simulink model "MPC_test_SG"  (R2024b)
settings: Solver=FixedStepAuto  StartTime=0.0  StopTime=20  FixedStep=0.02  RelTol=1e-3
values from neighbouring files (symbols this model uses):
  Eff = fit(Js, Effs, 'poly9')    [SG01_Flight_Dynamics.m]    (also in SG01_Flight_Dynamics_original.m)
  T = rho*(Rpms_propeller/60)^2*diam^4*kt    [SG01_Flight_Dynamics.m]    (also in SG01_Flight_Dynamics_original.m)
undefined symbols (not defined in the file or in its folder): initial_P, initial_Pitch, initial_Q, initial_R, initial_ROLL, initial_uspeed, initial_vspeed, initial_wspeed, initial_YAW, initial_Z
libraries: mpclib x1, slpidlib x1
settings Model: Creator=Basile  LastModifiedBy=ricar
settings SolverCC: ConcurrentTasks=on  ZeroCrossAlgorithm=Adaptive  AlgebraicLoopSolver=TrustRegion  PositivePriorityOrder=on
settings DataIOCC: ExternalInput=getinputstruct(op_trim1)  InitialState=getstatestruct(op_trim1)  SaveOutput=off  DSMLogging=off  SaveTime=off  ReturnWorkspaceOutputs=off
settings OptimizationCC: BlockReduction=off  DefaultParameterBehavior=Inlined  UseDivisionForNetSlopeComputation=on  UseFloatMulNetSlope=on  OptimizeBlockIOStorage=off  BufferReuse=off  PassReuseOutputArgsThreshold=0  EfficientFloat2IntCast=on  OptimizeBlockOrder=speed  DifferentSizesBufferReuse=on
settings DebuggingCC: InheritedTsInSrcMsg=none  TasksWithSamePriorityMsg=none  ParameterTunabilityLossMsg=error  UniqueDataStoreMsg=error  ArithmeticOperatorsInVariantConditions=warning
settings HardwareCC: ProdBitPerLong=64  ProdLongLongMode=on  ProdHWDeviceType=Intel->x86-64 (Linux 64)
settings ModelReferenceCC: EnableRefExpFcnMdlSchedulingChecks=on
settings SFSimCC: SimUseLocalCustomCode=off  MATLABDynamicMemAlloc=off  CustomCodeUndefinedFunction=UseInterfaceOnly
settings RTWCC: Description=Simulink Real-Time  SystemTargetFile=slrealtime.tlc  TemplateMakefile=slrealtime_default_tmf  GenerateReport=on  RTWUseLocalCustomCode=off  Toolchain=Simulink Real-Time Toolchain  BuildConfiguration=Faster Runs  LaunchReport=on  CodeExecutionProfiling=on  TargetLang=C++  GPUComputeCapability=3.5  DLArmComputeVersion=19.05
settings CodeAppCC: ForceParamTrailComments=on  OperatorAnnotations=on
settings SimulinkRealTimeTargetCC: InstructionSetFMA=off  LogToMDFFile=off

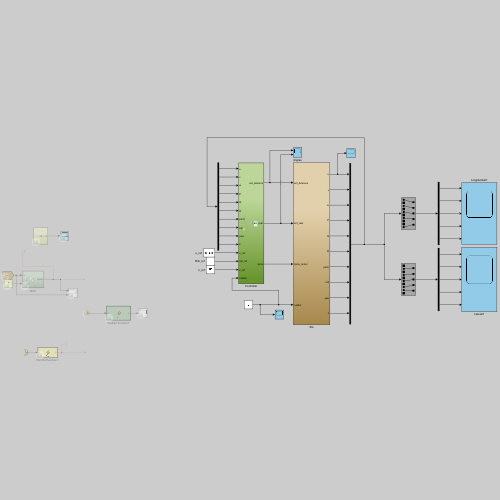
[thumbnail: Simulink's stored preview of the top-level diagram]
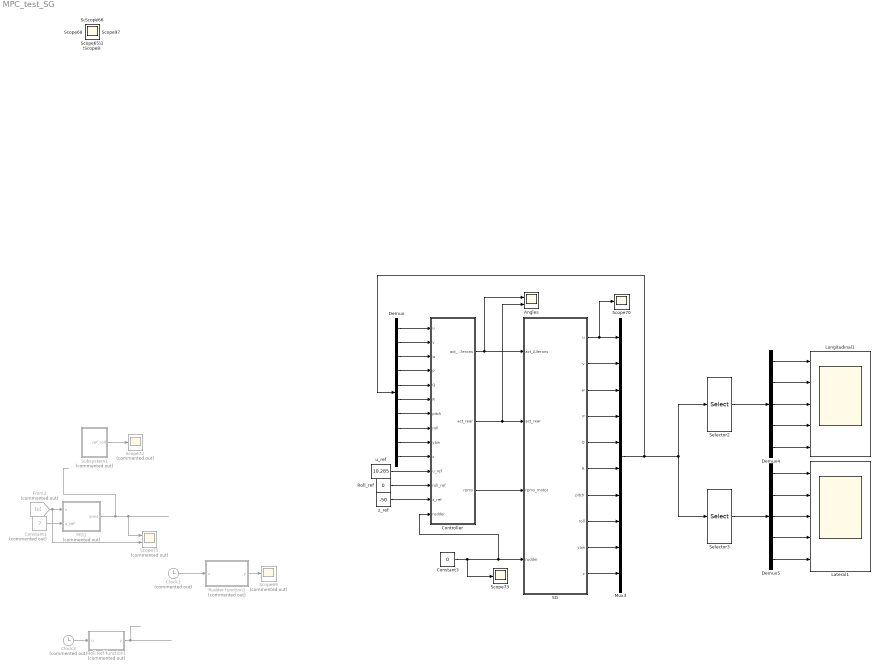
== system MPC_test_SG ==
  Angles : Scope  NumInputPorts=2
  Clock2 : Clock  Commented=on
  Clock3 : Clock  Commented=on
  Constant1 : Constant  Commented=on  Value=7
  Constant3 : Constant  Value=0
  Controller : Subsystem
  Demux : Demux  Outputs=10
  Demux4 : Demux  Outputs=5
  Demux5 : Demux  Outputs=5
  From2 : From  Commented=on  GotoTag=u
  Lateral1 : Scope  NumInputPorts=5
  Longitudinal1 : Scope  NumInputPorts=5
  Mux3 : Mux  Inputs=10
  PID1 : Subsystem  Commented=on
  Roll Ref function1 : MATLAB Function  Commented=on  TreatAsAtomicUnit=on
  Roll_ref : Constant  Value=0
  Rudder function1 : MATLAB Function  Commented=on  TreatAsAtomicUnit=on
  SG : Subsystem
  Scope69 : Scope  Commented=on
  Scope{,1..68,70,73} (71 alike) : Scope
  Scope72 : Scope  Commented=on
  Scope75 : Scope  Commented=on  NumInputPorts=2
  Selector2 : Selector  InputPortWidth=10  IndexOptions=Index vector (dialog)  Indices=[1 3 5 7 10]  OutputSizes=1
  Selector3 : Selector  InputPortWidth=10  IndexOptions=Index vector (dialog)  Indices=[2 4 6 8 9]  OutputSizes=1
  Subsystem1 : Subsystem  Commented=on
  u_ref : Constant  Value=10.285
  z_ref : Constant  Value=-50
  wires:
  SG/5(Q) -> Mux3/5
  SG/6(R) -> Mux3/6
  SG/7(pitch) -> Mux3/7
  Roll Ref function1/1(y) -> ?
  Rudder function1/1(y) -> Scope69/1
  Demux/9 -> Controller/9(yaw)
  Demux/3 -> Controller/3(w)
  Demux/8 -> Controller/8(roll)
  Demux/6 -> Controller/6(R)
  Demux/7 -> Controller/7(pitch)
  SG/10(z) -> Mux3/10
  Demux/2 -> Controller/2(v)
  Demux/5 -> Controller/5(Q)
  SG/4(P) -> Mux3/4
  SG/8(roll) -> Mux3/8
  Demux5/3 -> Lateral1/3
  Demux/10 -> Controller/10(z)
  Roll_ref/1 -> Controller/12(roll_ref)
  Subsystem1/1(ref_roll) -> Scope72/1
  Controller/2(act_rear) -> SG/2(act_rear), Angles/2
  Demux5/4 -> Lateral1/4
  Clock2/1 -> Rudder function1/1(u)
  Demux/4 -> Controller/4(P)
  Selector2/1 -> Demux4/1
  Mux3/1 -> Demux/1, Selector2/1, Selector3/1
  Clock3/1 -> Roll Ref function1/1(u)
  Selector3/1 -> Demux5/1
  Constant3/1 -> Controller/14(rudder), SG/4(rudder), Scope73/1
  Demux5/2 -> Lateral1/2
  Demux4/1 -> Longitudinal1/1
  Demux/1 -> Controller/1(u)
  Controller/1(act_ailerons) -> SG/1(act_Ailerons), Angles/1
  Demux5/5 -> Lateral1/5
  Demux5/1 -> Lateral1/1
  SG/1(u) -> Scope70/1, Mux3/1
  SG/9(yaw) -> Mux3/9
  Demux4/2 -> Longitudinal1/2
  Demux4/4 -> Longitudinal1/4
  z_ref/1 -> Controller/13(z_ref)
  Demux4/3 -> Longitudinal1/3
  SG/3(w) -> Mux3/3
  SG/2(v) -> Mux3/2
  Demux4/5 -> Longitudinal1/5
  Constant1/1 -> PID1/2(u_ref)
  PID1/1(rpms) -> Scope75/1
  From2/1 -> Scope75/2, PID1/1(u)
  u_ref/1 -> Controller/11(u_ref)
  Controller/3(rpms) -> SG/3(rpms_motor)

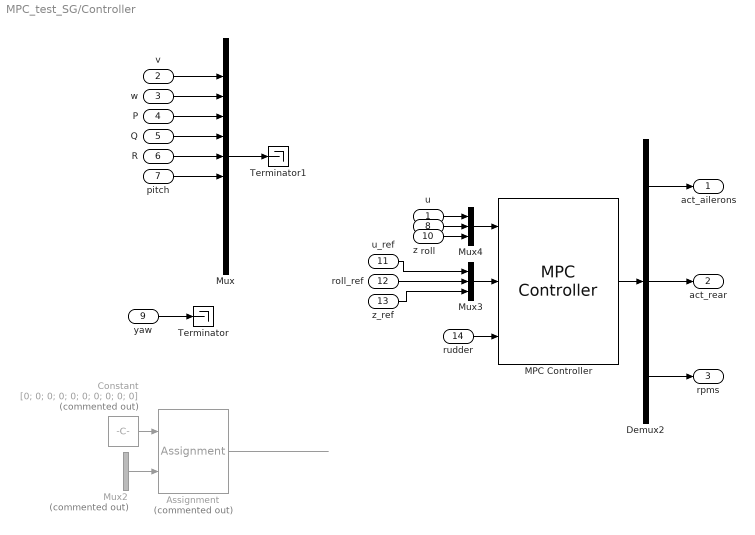
== system MPC_test_SG/Controller ==
  u : Inport
  v : Inport  Port=2
  w : Inport  Port=3
  P : Inport  Port=4
  Q : Inport  Port=5
  R : Inport  Port=6
  pitch : Inport  Port=7
  roll : Inport  Port=8
  yaw : Inport  Port=9
  z : Inport  Port=10
  u_ref : Inport  Port=11
  roll_ref : Inport  Port=12
  z_ref : Inport  Port=13
  rudder : Inport  Port=14
  Assignment : Assignment  Commented=on  DiagnosticForDimensions=Warning  IndexOptions=Index vector (dialog)  Indices=[1 10]  OutputSizes=1
  Constant : Constant  Commented=on  Value=[0; 0; 0; 0; 0; 0; 0; 0; 0; 0]
  Demux2 : Demux  Outputs=3
  MPC Controller : mpclib/MPC Controller  SCDEnableBlockLinearizationSpecification=on  mpcobj=mpcobj  is_multiple=0  enable_value=0  return_u0=off  updateMPCinCallerWorkspace=on  md_inport=on  mv_inport=off  uref_inport=off  return_cost=off  return_mvseq=off  return_qpstatus=off  return_xseq=off  return_state=off  return_ovseq=off  state_inport=off  umin_inport=off  umax_inport=off  ymin_inport=off  ymax_inport=off  cc_inport=off  ywt_inport=off  uwt_inport=off  duwt_inport=off  rhoeps_inport=off  pm_inport=off  MaximumP=10  HorizonChoice=FixedHorizon  n_ts=0.02  n_p=10  n_mv=3  n_md=1  n_ud=0  n_mo=3  n_uo=0  BlockDataType=double  SampleTimeInherited=off  switch_inport=off
  Mux : Mux  Inputs=11
  Mux2 : Mux  Commented=on  Inputs=2
  Mux3 : Mux  Inputs=3
  Mux4 : Mux  Inputs=3
  Terminator : Terminator
  Terminator1 : Terminator
  act_ailerons : Outport
  act_rear : Outport  Port=2
  rpms : Outport  Port=3
  wires:
  MPC Controller/1 -> Demux2/1
  Demux2/2 -> act_rear/1
  Demux2/1 -> act_ailerons/1
  Assignment/1 -> ?
  Constant/1 -> Assignment/1
  Mux2/1 -> Assignment/2
  yaw/1 -> Terminator/1
  R/1 -> Mux/6
  pitch/1 -> Mux/7
  Q/1 -> Mux/5
  P/1 -> Mux/4
  v/1 -> Mux/2
  w/1 -> Mux/3
  z/1 -> Mux4/3
  Mux4/1 -> MPC Controller/1
  roll/1 -> Mux4/2
  Mux/1 -> Terminator1/1
  Demux2/3 -> rpms/1
  Mux3/1 -> MPC Controller/2
  z_ref/1 -> Mux3/3
  roll_ref/1 -> Mux3/2
  u/1 -> Mux4/1
  rudder/1 -> MPC Controller/3
  u_ref/1 -> Mux3/1

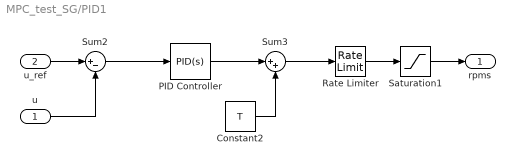
== system MPC_test_SG/PID1 ==
  u : Inport
  u_ref : Inport  Port=2
  Constant2 : Constant  Value=T
  PID Controller : slpidlib/PID Controller  Controller=PID  Form=Parallel  TimeDomain=Continuous-time  UseExternalTs=off  SampleTime=-1  IntegratorMethod=Forward Euler  FilterMethod=Forward Euler  ControllerParametersSource=internal  P=1000  I=10  UseKiTs=off  D=0  UseExternalDerivativeSource=off  N=100  UseFilter=on  TunerSelectOption=Transfer Function Based (PID Tuner App)  InitialConditionSource=internal  InitialConditionForIntegrator=0  InitialConditionForFilter=0  DifferentiatorICPrevScaledInput=0  ExternalReset=none  TrackingMode=off  Kt=1  LimitOutput=off  SatLimitsSource=internal  UpperSaturationLimit=inf  LowerSaturationLimit=-inf  LinearizeAsGain=on  AntiWindupMode=none  Kb=1  LimitIntegrator=off  UpperIntegratorSaturationLimit=inf  LowerIntegratorSaturationLimit=-inf  POutMin=[]  POutMax=[]  IOutMin=[]  IOutMax=[]  DOutMin=[]  DOutMax=[]  NOutMin=[]  NOutMax=[]  SumOutMin=[]  SumOutMax=[]  SaturationOutMin=[]  SaturationOutMax=[]  PParamMin=[]  PParamMax=[]  IParamMin=[]  IParamMax=[]  DParamMin=[]  DParamMax=[]  NParamMin=[]  NParamMax=[]  KbParamMin=[]  KbParamMax=[]  KtParamMin=[]  KtParamMax=[]  KbOutMin=[]  KbOutMax=[]  KtOutMin=[]  KtOutMax=[]  IntegratorOutMin=[]  IntegratorOutMax=[]  FilterOutMin=[]  FilterOutMax=[]  SumI1OutMin=[]  SumI1OutMax=[]  SumI2OutMin=[]  SumI2OutMax=[]  SumI3OutMin=[]  SumI3OutMax=[]  SumI4OutMin=[]  SumI4OutMax=[]  SumDOutMin=[]  SumDOutMax=[]  DifferentiatorOutMin=[]  DifferentiatorOutMax=[]  FilterDiffOutCoefMin=[]  FilterDiffOutCoefMax=[]  ReciprocalOutMin=[]  ReciprocalOutMax=[]  SumDenOutMin=[]  SumDenOutMax=[]  SumNumOutMin=[]  SumNumOutMax=[]  DivideOutMin=[]  DivideOutMax=[]  UdiffTsProdOutMin=[]  UdiffTsProdOutMax=[]  NTsProdOutMin=[]  NTsProdOutMax=[]  UintegralTsProdOutMin=[]  UintegralTsProdOutMax=[]  UngainTsProdOutMin=[]  UngainTsProdOutMax=[]  ClampingZeroOutDataTypeStr=Inherit: Inherit via back propagation  ClampingZeroOutMin=[]  ClampingZeroOutMax=[]  FilterDenConstantOutDataTypeStr=Inherit: Inherit via back propagation  FilterDenConstantOutMin=[]  FilterDenConstantOutMax=[]  PCopyOutDataTypeStr=Inherit: Inherit via back propagation  PCopyOutMin=[]  PCopyOutMax=[]  NCopyOutDataTypeStr=Inherit: Inherit via back propagation  NCopyOutMin=[]  NCopyOutMax=[]  IntegratorContinuousStateAttributes=''  IntegratorStateMustResolveToSignalObject=off  IntegratorRTWStateStorageClass=Auto  FilterContinuousStateAttributes=''  FilterStateMustResolveToSignalObject=off  FilterRTWStateStorageClass=Auto  ParallelPVariant=InternalParameters  IdealPVariant=Disabled  IVariant=InternalParameters  DVariant=InternalParameters  IntegratorVariant=Continuous  SatVariant=Disabled  AWVariant=Passthrough  PCopyVariant=Disabled  TRVariant=Disabled  FdbkBlocksVariant=Forward  IdealPFdbkVariant=Disabled  SatFdbkVariant=Disabled  DerivativeFilterVariant=ContFilter  NVariant=InternalParameters  NCopyVariant=Disabled  FilterICVariant=InternalICsFilter  IntegratorICVariant=InternalICs  ExternalResetVariant=Disabled  TRSumVariant=Passthrough  SumFdbkVariant=Disabled  SumVariant=Sum_PID  TsampFilterVariant=InternalTs  TsampNgainVariant=Passthrough  TsampIntegralVariant=Disabled_SignalSpec  ExternalSaturationOutDataTypeStr=Inherit: Same as second input  DerivativeSourceVariant=ErrorSignal
  Rate Limiter : RateLimiter  RisingSlewLimit=1000  FallingSlewLimit=-1000  SampleTimeMode=inherited  InitialCondition=T
  Saturation1 : Saturate  UpperLimit=9000
  Sum2 : Sum  Inputs=|+-
  Sum3 : Sum  Inputs=|++
  rpms : Outport
  wires:
  Rate Limiter/1 -> Saturation1/1
  u/1 -> Sum2/2
  Sum3/1 -> Rate Limiter/1
  Sum2/1 -> PID Controller/1
  u_ref/1 -> Sum2/1
  Constant2/1 -> Sum3/2
  Saturation1/1 -> rpms/1
  PID Controller/1 -> Sum3/1

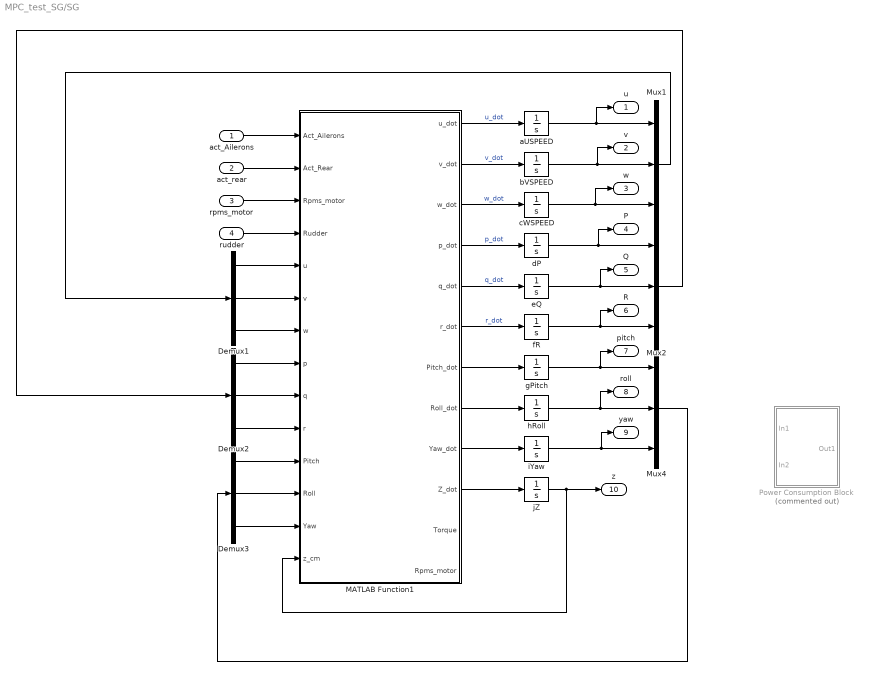
== system MPC_test_SG/SG ==
  act_Ailerons : Inport
  act_rear : Inport  Port=2
  rpms_motor : Inport  Port=3
  rudder : Inport  Port=4
  Demux1 : Demux  Outputs=3
  Demux2 : Demux  Outputs=3
  Demux3 : Demux  Outputs=3
  MATLAB Function1 : MATLAB Function  TreatAsAtomicUnit=on
  Mux1 : Mux  Inputs=3
  Mux2 : Mux  Inputs=3
  Mux4 : Mux  Inputs=3
  Power Consumption Block : Subsystem  Commented=on
  aUSPEED : Integrator  InitialCondition=initial_uspeed
  bVSPEED : Integrator  InitialCondition=initial_vspeed
  cWSPEED : Integrator  InitialCondition=initial_wspeed
  dP : Integrator  InitialCondition=initial_P
  eQ : Integrator  InitialCondition=initial_Q
  fR : Integrator  InitialCondition=initial_R
  gPitch : Integrator  InitialCondition=initial_Pitch
  hRoll : Integrator  InitialCondition=initial_ROLL
  iYaw : Integrator  InitialCondition=initial_YAW
  jZ : Integrator  InitialCondition=initial_Z
  u : Outport
  v : Outport  Port=2
  w : Outport  Port=3
  P : Outport  Port=4
  Q : Outport  Port=5
  R : Outport  Port=6
  pitch : Outport  Port=7
  roll : Outport  Port=8
  yaw : Outport  Port=9
  z : Outport  Port=10
  wires:
  eQ/1 -> Q/1, Mux2/2
  rpms_motor/1 -> MATLAB Function1/3("Rpms_motor ")
  gPitch/1 -> pitch/1, Mux4/1
  hRoll/1 -> roll/1, Mux4/2
  act_rear/1 -> MATLAB Function1/2(Act_Rear)
  MATLAB Function1/10(Z_dot) -> jZ/1
  cWSPEED/1 -> w/1, Mux1/3
  dP/1 -> P/1, Mux2/1
  iYaw/1 -> yaw/1, Mux4/3
  MATLAB Function1/1(u_dot) -> aUSPEED/1  "u_dot"
  rudder/1 -> MATLAB Function1/4(Rudder)
  jZ/1 -> z/1, MATLAB Function1/14(z_cm)
  Demux2/2 -> MATLAB Function1/9(q)
  MATLAB Function1/3(w_dot) -> cWSPEED/1  "w_dot"
  Mux2/1 -> Demux2/1
  MATLAB Function1/4(p_dot) -> dP/1  "p_dot"
  Demux1/3 -> MATLAB Function1/7(w)
  MATLAB Function1/9(Yaw_dot) -> iYaw/1
  Demux1/2 -> MATLAB Function1/6(v)
  MATLAB Function1/2(v_dot) -> bVSPEED/1  "v_dot"
  MATLAB Function1/8(Roll_dot) -> hRoll/1
  Mux1/1 -> Demux1/1
  fR/1 -> R/1, Mux2/3
  Demux1/1 -> MATLAB Function1/5(u)
  MATLAB Function1/6(r_dot) -> fR/1  "r_dot"
  Demux3/1 -> MATLAB Function1/11(Pitch)
  bVSPEED/1 -> v/1, Mux1/2
  act_Ailerons/1 -> MATLAB Function1/1(Act_Ailerons)
  Demux2/1 -> MATLAB Function1/8(p)
  Demux3/2 -> MATLAB Function1/12(Roll)
  Demux3/3 -> MATLAB Function1/13(Yaw)
  Mux4/1 -> Demux3/1
  MATLAB Function1/5(q_dot) -> eQ/1  "q_dot"
  MATLAB Function1/7(Pitch_dot) -> gPitch/1
  Demux2/3 -> MATLAB Function1/10(r)
  aUSPEED/1 -> u/1, Mux1/1

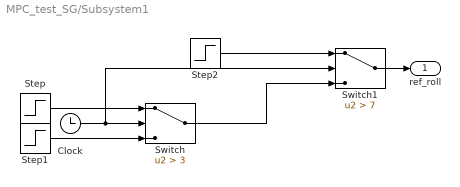
== system MPC_test_SG/Subsystem1 ==
  Clock : Clock
  Step : Step  Time=4  Before=11  After=-11  SampleTime=0
  Step1 : Step  After=11  SampleTime=0
  Step2 : Step  Time=7  Before=-11  After=0  SampleTime=0
  Switch : Switch  Criteria=u2 > Threshold  Threshold=3  SaturateOnIntegerOverflow=off  InputSameDT=off
  Switch1 : Switch  Criteria=u2 > Threshold  Threshold=7  SaturateOnIntegerOverflow=off  InputSameDT=off
  ref_roll : Outport
  wires:
  Switch/1 -> Switch1/3
  Step1/1 -> Switch/3
  Step/1 -> Switch/1
  Clock/1 -> Switch1/2, Switch/2
  Switch1/1 -> ref_roll/1
  Step2/1 -> Switch1/1

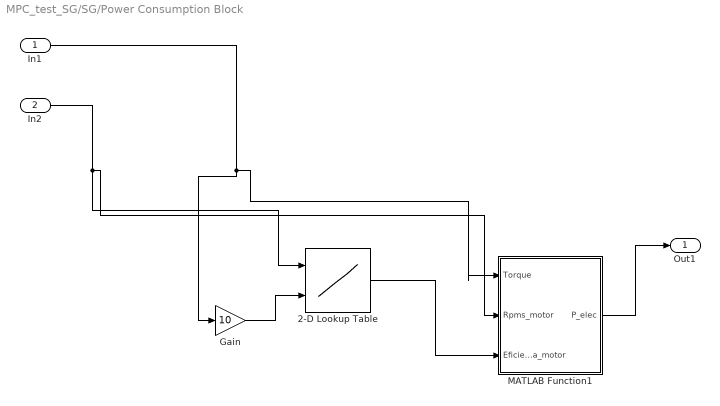
== system MPC_test_SG/SG/Power Consumption Block ==
  In1 : Inport
  In2 : Inport  Port=2
  2-D Lookup Table : Lookup_n-D  BreakpointsForDimension1=[1:6000]  BreakpointsForDimension2=[1:140]  Table=Eff  InternalRulePriority=Speed  RndMeth=Simplest
      settings: InputPortMap=u0,u1
  Gain : Gain  Gain=10
  MATLAB Function1 : MATLAB Function  TreatAsAtomicUnit=on
  Out1 : Outport
  wires:
  In2/1 -> 2-D Lookup Table/1, MATLAB Function1/2(Rpms_motor)
  MATLAB Function1/1(P_elec) -> Out1/1
  In1/1 -> Gain/1, MATLAB Function1/1(Torque)
  Gain/1 -> 2-D Lookup Table/2
  2-D Lookup Table/1 -> MATLAB Function1/3(Eficiencia_motor)

== matlab function MPC_test_SG/SG/MATLAB Function1 ==
  data: Act_Ailerons input; Act_Rear input; Rpms_motor input; Rudder input; u input; u_dot output; v input; w input; p input; q input; r input; Pitch input; Roll input; Yaw input; z_cm input; v_dot output; w_dot output; p_dot output; q_dot output; r_dot output; Pitch_dot output; Roll_dot output; Yaw_dot output; Z_dot output; Torque output; Rpms_motor output
function [u_dot,v_dot,w_dot,p_dot,q_dot,r_dot,Pitch_dot,Roll_dot,Yaw_dot,Z_dot,Torque,Rpms_motor] = SG01_Flight_Dynamics(Act_Ailerons,Act_Rear,Rpms_motor, Rudder,u,v,w,p,q,r,Pitch,Roll,Yaw,z_cm)

% Modelo Dinâmico do SG01, recebendo o estado do sistema ele retorna as
% derivadas das velocidades da "embarcação"

%%% CONSTANTES %%%

struts = 1;
wponto = 0;

g = 9.81; % Gravidade (m/s^2)
rho= 1026.00; % Densidade água salgada (kg/m^3)
mu= 1.14E-3; % Coef. viscosidade dinâmica água salgada (Pa*s)
m = 2000; % Massa da "embarcação" (Kg)
Ixx = 294.2;
Iyy = 1.788e+04; % Momentos de Inércia
Izz = 1.759e+04;
Ixz = 404.7; % Produto de Inércia relevante
b = 2.400; % Span da Asa
c = 0.30988; % Corda média da Asa
S = 0.68757769; % Área da Asa
S_t = 0.20158673; % Área Elevator

if struts == 1 % struts estendidas, distancia submersa de strut
    z_struts = 1360 - z_cm/10; % estimativa muito rough
else
    z_struts = 0; % struts não estendidas INCLUIR AQUI TAMBÉM DIFERENTES DERIVADAS NO FUTURO
end


%%% DISTÂNCIAS %%% Esta secção deixou de ser necessária, acredito eu
x_cg_asas = 0.771; %centroide assumindo asa de tras semi eliptica e frente eliptica num referencial com origem a 20cm do leading edge da asa apontado para a cauda
X_CG_ASASRUDDERSTRUTS = (x_cg_asas*(S_t+S)-100*z_struts*2.825)/(S_t+S+100*z_struts); %X do CG das asa + rudder + struts no referencial com origem no meio da asa da frente CUIDADO COM O Z_STRUTS, que esta em mm
Z_CG_ASASRUDDERSTRUTS = (3*0.5*z_struts*100*z_struts)/(S_t+S+100*z_struts);
dist_CGSG_CGASAS_X = 3.715+X_CG_ASASRUDDERSTRUTS-3.964;
dist_CGSG_CGASAS_Y = 0; %idealmente
dist_CGSG_CGASAS_Z = z_struts + 1;

%%% Derivadas de estabilidade e controlo %%%
V = 10.28;
u0 = cos(deg2rad(-3.558))*V;
w0 = sin(deg2rad(-3.558))*V;
deltau = u - u0;
deltaw = w - w0;
deltaAct_Rear = Act_Rear - 4;
teta0 = -3.558;
Cw0 = (m*g*cos(teta0))/(0.5*rho*(u0^2)*S);
Cd1 = 0.015;

CXu = -0.02440;
CZu = -0.00701;
CMu = 0.08341;
CXa = 0.22694;
CLa = 5.93757;
CMa = -9.37193;
CXwponto = 0;
CLwponto = 0; % Não tenho como saber ainda
CMwponto = 0;
CXq = -0.31325;
CLq = 42.62028;
CMq = -319.07598;
CYb = -0.10815;
Clb = 0.11373;
CNb = 0.15492;
CYp = 0.18263;
Clp = -0.72524;
CNp = -0.33702;
CYr = 0.32068;
Clr = -0.22191;
CNr = -0.45556;
CXd_a = -0.00673;
CYd_a = 0.02042;
CZd_a = -0.26237;
Cld_a = 0.20542;
CMd_a = 0.06255;
CNd_a = -0.01074;
CXd_t = -0.01195;
CYd_t = 0; % meti a 0 porque não faz sentido
CZd_t = -1.20579;
Cld_t = 0;
CMd_t = -13.51024;
CNd_t = 0;
CXd_r = -0.01692;
CYd_r = 0.08540;
CZd_r = -0.35782;
Cld_r = -0.19211;
CMd_r = 0.13566;
CNd_r = -0.12412;

%%% DERIVADAS DIMENSIONAIS DE ESTABILIDADE %%

beta = asin(min(u/V,1));
alpha = atan(w/V);

Xu = rho*u0*S*sin(teta0)*Cw0 + 0.5*rho*S*u0*CXu;
Zu = -rho*u0*S*cos(teta0)*Cw0 + 0.5*rho*S*u0*CZu;
Mu = 0.5*rho*S*u0*c*CMu;
du = [Xu ; Zu ; Mu];

Xw = 0.5*rho*S*u0*CXa;
CZa = -(CLa + Cd1);
Zw = 0.5*rho*S*u0*CZa;
Mw = 0.5*rho*S*u0*CMa;
dw = [Xw ; Zw ; Mw];

Xwponto = 0.25*rho*S*c*CXwponto;
CZwponto = -CLwponto;
Zwponto = 0.25*rho*S*c*CZwponto;
Mwponto = 0.25*rho*S*c*c*CMwponto;
dwponto = [Xwponto ; Zwponto ; Mwponto];

Xq = 0.25*rho*S*u0*c*CXq;
CZq = -CLq;
Zq = 0.25*rho*S*u0*c*CZq;
Mq = 0.25*rho*S*u0*c*c*CMq;
dq = [Xq ; Zq ; Mq];

Yv = 0.25*rho*S*u0*CYb;
Lv = 0.5*rho*S*u0*beta*Clb;
Nv = 0.5*rho*S*u0*beta*CNb;
dv = [Yv ; Lv ; Nv];

Yp = 0.25*rho*u0*S*beta*CYp;
Lp = 0.25*rho*u0*S*beta*beta*Clp;
Np = 0.25*rho*u0*S*beta*beta*CNp;
dp = [Yp ; Lp ; Np];

Yr = 0.25*rho*S*u0*beta*CYr;
Lr = 0.25*rho*S*u0*beta*beta*Clr;
Nr = 0.25*rho*S*u0*beta*beta*CNr;
dr = [Yr ; Lr ; Nr];

%%% DERIVADAS DIMENSIONAIS CONTRLOLO EM RADIANOS%

Act_Ailerons = deg2rad(Act_Ailerons);
Act_Rear = deg2rad(Act_Rear);
Rudder = deg2rad(Rudder);

Xd_a = 0.5*rho*u0*u0*S*CXd_a;
Yd_a = 0.5*rho*u0*u0*S*CYd_a;
Zd_a = 0.5*rho*u0*u0*S*CZd_a;
Ld_a = 0.5*rho*u0*u0*S*beta*Cld_a;
Md_a = 0.5*rho*u0*u0*S*c*CMd_a;
Nd_a = 0.5*rho*u0*u0*S*beta*CNd_a;

Xd_t = 0.5*rho*u0*u0*S*CXd_t;
Yd_t = 0.5*rho*u0*u0*S*CYd_t;
Zd_t = 0.5*rho*u0*u0*S*CZd_t;
Ld_t = 0.5*rho*u0*u0*S*beta*Cld_t;
Md_t = 0.5*rho*u0*u0*S*c*CMd_t;
Nd_t = 0.5*rho*u0*u0*S*beta*CNd_t;

Xd_r = 0.5*rho*u0*u0*S*CXd_r;
Yd_r = 0.5*rho*u0*u0*S*CYd_r;
Zd_r = 0.5*rho*u0*u0*S*CZd_r;
Ld_r = 0.5*rho*u0*u0*S*beta*Cld_r;
Md_r = 0.5*rho*u0*u0*S*c*CMd_r;
Nd_r = 0.5*rho*u0*u0*S*beta*CNd_r;

%%% ALGURES CONDIÇÃO DE VENTILAÇÃO %%%

%%% THRUST %%%

Rpms_propeller = Rpms_motor/3;
diam = 0.335;

% Coefficients for KT 
KT_p1 = -39.575;
KT_p2 = 296.698;
KT_p3 = -977.420;
KT_p4 = 1855.793;
KT_p5 = -2236.302;
KT_p6 = 1772.128;
KT_p7 = -922.459;
KT_p8 = 303.597;
KT_p9 = -57.450;
KT_p10 = 5.070;

% KT function 
KT = @(x) KT_p1*x.^9 + KT_p2*x.^8 + KT_p3*x.^7 + KT_p4*x.^6 + KT_p5*x.^5 + KT_p6*x.^4 + KT_p7*x.^3 + KT_p8*x.^2 + KT_p9*x + KT_p10;

 
% Coefficients for kq 
Kq_p1 = 2.787;
Kq_p2 = -23.468;
Kq_p3 = 85.726;
Kq_p4 = -178.762;
Kq_p5 = 234.931;
Kq_p6 = -202.035;
Kq_p7 = 113.776;
Kq_p8 = -40.505;
Kq_p9 = 8.257;
Kq_p10 = -0.689;

% Kq function 
Kq = @(x) Kq_p1*x.^9 + Kq_p2*x.^8 + Kq_p3*x.^7 + Kq_p4*x.^6 + Kq_p5*x.^5 + Kq_p6*x.^4 + Kq_p7*x.^3 + Kq_p8*x.^2 + Kq_p9*x + Kq_p10;

 
Eff_p1 = -8627.603;
Eff_p2 = 61047.137;
Eff_p3 = -190004.847;
Eff_p4 = 341275.626;
Eff_p5 = -389694.487;
Eff_p6 = 293275.528;
Eff_p7 = -145425.793;
Eff_p8 = 45806.430;
Eff_p9 = -8313.959;
Eff_p10 = 662.694;
% Eff function 
Eff = @(x) Eff_p1*x.^9 + Eff_p2*x.^8 + Eff_p3*x.^7 + Eff_p4*x.^6 + Eff_p5*x.^5 + Eff_p6*x.^4 + Eff_p7*x.^3 + Eff_p8*x.^2 + Eff_p9*x + Eff_p10;

js = 60*V/(Rpms_propeller*diam);

kq = Kq(js);
kt = KT(js);
eff = Eff(js);

T = rho*(Rpms_propeller/60)^2*diam^4*kt;
P_propeller = T*V/eff;

%Calculate Power usage
P_mec=P_propeller/0.8;
Torque=P_mec/(Rpms_motor*2*pi/60);

%%% SOMATÓRIO %%%

X = du(1)*deltau + dw(1)*deltaw + dwponto(1)*wponto + dq(1)*q + Xd_a*Act_Ailerons + Xd_t*deltaAct_Rear + Xd_r*Rudder;
Y = dv(1)*v + dp(1)*p + dr(1)*r + Yd_a*Act_Ailerons + Yd_t*Act_Rear + Yd_r*Rudder;
Z = du(2)*deltau + dw(2)*deltaw + dwponto(2)*wponto + dq(2)*q + Zd_a*Act_Ailerons + Zd_t*deltaAct_Rear + Zd_r*Rudder;
L = dv(2)*v + dp(2)*p + dr(2)*r + Ld_a*Act_Ailerons + Ld_t*Act_Rear + Ld_r*Rudder;
M = du(3)*deltau + dw(3)*deltaw + dwponto(3)*wponto + dq(3)*q + Md_a*Act_Ailerons + Md_t*deltaAct_Rear + Md_r*Rudder;
N = dv(3)*v + dp(3)*p + dr(3)*r + Nd_a*Act_Ailerons + Nd_t*Act_Rear + Nd_r*Rudder;

%d = [dist_CGSG_CGASAS_X ; dist_CGSG_CGASAS_Y ; dist_CGSG_CGASAS_Z];
F = [X + T ; Y ; Z];
%M_1 = cross(d,F); não é necessário porque forças já estão no CG

M_2 = [L ; M ; N];

M_T = [0 ; 2.6 * T; 0]; % Momento só do Thrust, confia
Tau = M_2 + M_T; % Momentos livres + Momentos das Forças no CG do SG


%%% DERIVADAS %%%

R = [cosd(Pitch)*cosd(Yaw) cosd(Pitch)*sind(Yaw) -sind(Pitch);
    sind(Roll)*sind(Pitch)*cosd(Yaw)-cosd(Roll)*sind(Yaw) sind(Roll)*sind(Pitch)*sind(Yaw)+cosd(Roll)*cosd(Yaw) sind(Roll)*cosd(Pitch);
    cosd(Roll)*sind(Pitch)*cosd(Yaw)+sind(Roll)*sind(Yaw) cosd(Roll)*sind(Pitch)*sind(Yaw)-sind(Roll)*cosd(Yaw) cosd(Roll)*cosd(Pitch)]; % MATRIZ DE TRANSFERÊNCIA DE REFERENCIAL

%Balance of forces
p = p*pi/180;
q = q*pi/180;
r = r*pi/180;
ww = [p;q;r];

%W_inertial = m*g*[0;0;1];
W_inertial = 0;

uvw_dot = (F + R*W_inertial)/m - cross(ww, [u;v;w]);
VI_dot = R'*[u;v;w];

%Inertial angular velocities
Q = [1 sind(Roll)*tand(Pitch) cosd(Roll)*tand(Pitch);
     0 cosd(Roll) -sind(Roll);
     0 sind(Roll)/cosd(Pitch) cosd(Roll)/cosd(Pitch)];
eul = Q*ww;
Roll_dot = eul(1);
Pitch_dot = eul(2);
Yaw_dot = eul(3);

%Balance of moments

J = [Ixx 0 Ixz;
     0   Iyy 0;
     Ixz 0 Izz];
invJ = [-Izz/(Ixz^2 - Ixx*Izz),     0,  Ixz/(Ixz^2 - Ixx*Izz);
            0,                  1/Iyy,                      0;
       Ixz/(Ixz^2 - Ixx*Izz),     0,  -Ixx/(Ixz^2 - Ixx*Izz)];

wdot = invJ*(Tau - cross(ww,J*ww));

p_dot = wdot(1)*180/pi;
q_dot = wdot(2)*180/pi;
r_dot = wdot(3)*180/pi;

u_dot = uvw_dot(1);
v_dot = uvw_dot(2);
w_dot = uvw_dot(3);

Z_dot = VI_dot(3);
end

== matlab function MPC_test_SG/Roll Ref function1 ==
  data: u input; y output
function y = fcn(u)
t1 = 10;
t2 = 10.5;
t3 = 14.5;
t4 = 15;
t5 = 15;
t6 = 15;

v1 = 0;
v2 = 10;
v3 = 0;
v4 = 0;

if (u < t1)
    y = v1;
elseif (t1 <= u && u < t2)
    y = (v2-v1)/(t2-t1)*(u-t1) + v1;
elseif (t2 <= u && u < t3)
    y = v2;
elseif (t3 <= u && u < t4)
    y = (v3-v2)/(t4-t3)*(u-t3) + v2;
elseif (t4 <= u && u < t5)
    y = v3;
elseif (t5 <= u && u < t6)
    y = (v4-v3)/(t6-t5)*(u-t5) + v3;
else 
    y = v4;
end

end

== matlab function MPC_test_SG/Rudder function1 ==
  data: u input; y output
function y = fcn(u)
t1 = 5;
t2 = 5.5;
t3 = 9.5;
t4 = 10;
t5 = 10;
t6 = 10;

v1 = 0;
v2 = 15;
v3 = 0;
v4 = 0;

if (u < t1)
    y = v1;
elseif (t1 <= u && u < t2)
    y = (v2-v1)/(t2-t1)*(u-t1) + v1;
elseif (t2 <= u && u < t3)
    y = v2;
elseif (t3 <= u && u < t4)
    y = (v3-v2)/(t4-t3)*(u-t3) + v2;
elseif (t4 <= u && u < t5)
    y = v3;
elseif (t5 <= u && u < t6)
    y = (v4-v3)/(t6-t5)*(u-t5) + v3;
else 
    y = v4;
end

end

== matlab function MPC_test_SG/SG/Power Consumption Block/MATLAB Function1 ==
  data: Torque input; P_elec output; Rpms_motor input; Eficiencia_motor input
function P_elec = fcn(Torque,Rpms_motor,Eficiencia_motor)
P_mec = Torque*Rpms_motor*2*pi/60;
P_elec = P_mec/Eficiencia_motor;
